simulink model "Monitoring_R2017b"  (R2017b)
settings: Solver=FixedStepAuto  StartTime=0.0  StopTime=inf  FixedStep=0.01  RelTol=1e-3
values from neighbouring files (symbols this model uses):
  f = [0.01 0.0100092155052 0.0100184395029 0.010027672001 0.0100369130073 0.0100461625297 0.0100554205759 0.010064687154 0.0100739622716 0.0100832459368 0.0100925381573 0.010101838941 ... (10000 elements, 1x10000)]    [abc_ws.mat]    (also in kalmanSSHumInput.m = logspace(-2,2,1e4); tests_analysis.m = (1/dt)*(0:(L/2))/L)
libraries: instrumentlib x1
settings Model: Creator=guilherme  LastModifiedBy=leona

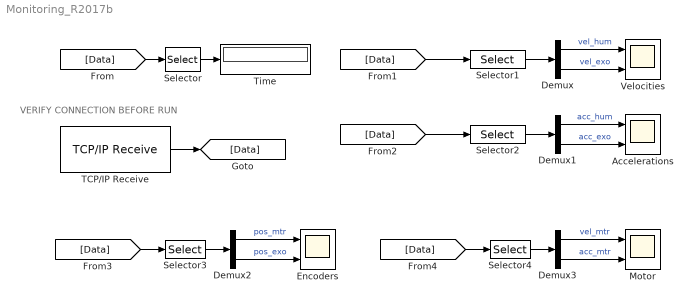
== system Monitoring_R2017b ==
  note: VERIFY CONNECTION BEFORE RUN
  Accelerations : Scope  NumInputPorts=2
  Demux{,1..3} (4 alike) : Demux  Outputs=2
  Encoders : Scope  NumInputPorts=2
  Motor : Scope  NumInputPorts=2
  Selector : Selector  InputPortWidth=9  IndexOptions=Index vector (dialog)  Indices=[1]  OutputSizes=1
  Selector1 : Selector  InputPortWidth=9  IndexOptions=Index vector (dialog)  Indices=[2 3]  OutputSizes=1
  Selector2 : Selector  InputPortWidth=9  IndexOptions=Index vector (dialog)  Indices=[4 5]  OutputSizes=1
  Selector3 : Selector  InputPortWidth=9  IndexOptions=Index vector (dialog)  Indices=[6 7]  OutputSizes=1
  Selector4 : Selector  InputPortWidth=9  IndexOptions=Index vector (dialog)  Indices=[8 9]  OutputSizes=1
  TCP/IP Receive : instrumentlib/TCP//IP Receive  Host=0.0.0.0  Port=2324  DataSize="[1  9]"  EnableBlockingMode=on  Timeout=10  SampleTime=0.01  DataType=single  ByteOrder=BigEndian  ASCIIFormatting=%f,  Terminator=LF
  Time : Display
  Velocities : Scope  NumInputPorts=2
  wires:
  Selector/1 -> Time/1
  Demux/1 -> Velocities/1  "vel_hum"
  Demux/2 -> Velocities/2  "vel_exo"
  Selector1/1 -> Demux/1
  Selector2/1 -> Demux1/1
  Demux1/2 -> Accelerations/2  "acc_exo"
  Demux1/1 -> Accelerations/1  "acc_hum"
  Demux2/1 -> Encoders/1  "pos_mtr"
  Demux2/2 -> Encoders/2  "pos_exo"
  Selector3/1 -> Demux2/1
  TCP/IP Receive/1 -> [Data]
  [Data] -> Selector/1
  [Data] -> Selector1/1
  [Data] -> Selector2/1
  [Data] -> Selector3/1
  [Data] -> Selector4/1
  Selector4/1 -> Demux3/1
  Demux3/2 -> Motor/2  "acc_mtr"
  Demux3/1 -> Motor/1  "vel_mtr"
